simulink model "modelo_f_nico_local"  (R2024b)
settings: Solver=ode15s  StartTime=0.0  StopTime=600  FixedStep=0.001  RelTol=1e-3
InitFcn:
  | clc
  | clear
  | close all
  | parametros
  | gain_CL
  | calculo_observador_carro
  | calculo_observador_izaje
values from neighbouring files (symbols this model uses):
  b_cx = 1e6    (= 1000000)    [parametros.m]
  b_cy = 1e7    (= 10000000)    [parametros.m]
  b_ha = -(J_hEq + (r_hd/(2*i_h))*m_l) * w_des_h*(1 + n_h + n_h^2) + b_hEq    [gain_CL.m]
  b_hb = 1e8    (= 100000000)    [parametros.m]
  b_hd = 8    [parametros.m]
  b_hm = 18    [parametros.m]
  b_t = 90    [parametros.m]
  b_ta = M_tEq*w_des_t*(1+n_t+n_t^2)-b_tEq    [gain_CL.m]
  b_tb = 5e6    (= 5000000)    [parametros.m]
  b_td = 1.8    [parametros.m]
  b_tm = 6    [parametros.m]
  b_tw = 3e3    (= 3000)    [parametros.m]
  b_wu = 150    [parametros.m]
  g = 9.80665    [parametros.m]
  H_c = 2.59    [parametros.m]
  i_h = 22    [parametros.m]
  i_t = 30    [parametros.m]
  J_hd_hEb = 3800    [parametros.m]
  J_hm_hb = 30    [parametros.m]
  J_td = 1200    [parametros.m]
  J_tm_tb = 7    [parametros.m]
  K_cy = 1.8e9    (= 1800000000)    [parametros.m]
  k_hsa = -(J_hEq + (r_hd/(2*i_h))*m_l) * w_des_h^2*(n_h + n_h^2 + n_h^3)    [gain_CL.m]
  k_hsia = -(J_hEq + (r_hd/(2*i_h))*m_l) * n_h^3 * w_des_h^3    [gain_CL.m]
  k_tsa = M_tEq*w_des_t^2*n_t*(1+n_t+n_t^2)    [gain_CL.m]
  k_tsia = M_tEq*w_des_t^3*n_t^3    [gain_CL.m]
  K_tw = 4.8e5    (= 480000)    [parametros.m]
  k_wu = 2.36e8    (= 236000000)    [parametros.m]
  l_h_max = Y_t0-y_h_min    (= 65)    [parametros.m]
  l_h_maxE = l_h_max+0.5    (= 65.5)    [parametros.m]
  l_h_min = Y_t0-y_h_max    (= 5)    [parametros.m]
  l_h_minE = l_h_min-0.5    (= 4.5)    [parametros.m]
  Lt = place(At', Ct', polos_deseados)'    [calculo_observador_carro.m]
  M_cmax = 50000    [parametros.m]
  M_cmin = 2000    [parametros.m]
  M_s = 15000    [parametros.m]
  M_t = 30000    [parametros.m]
  r_hd = 0.75    [parametros.m]
  r_td = 0.50    (= 0.5)    [parametros.m]
  T_hbMax = 5e4    (= 50000)    [parametros.m]
  T_hEbMax = 1.1e6    (= 1100000)    [parametros.m]
  T_hmMax = 2e4    (= 20000)    [parametros.m]
  T_s = 0.001    [parametros.m]
  T_tbMax = 5e3    (= 5000)    [parametros.m]
  T_tmMax = 4e3    (= 4000)    [parametros.m]
  tau_tm = 1e-3    (= 0.001)    [parametros.m]
  tau_wl = 1 / (2 * pi * 2)    (= 0.0795774715459)    [parametros.m]
  theta_hm0 = -l_h0*i_h*2/r_hd    (= -2229.33333333)    [parametros.m]
  theta_tm0 = (x_t0)*i_t/r_td    (= -900)    [parametros.m]
  v_h_max_noload = 3    [parametros.m]
  v_lx0 = 0    [parametros.m]
  v_ly0 = 0    [parametros.m]
  v_t0 = 0    [parametros.m]
  v_t_max = 4    [parametros.m]
  W_c = ctrb(A, B_c(:,1))    [CyO_carro.m]    (also in CyO_izaje.m; parametros.m = 2.44)
  w_hm0 = 0    [parametros.m]
  w_hm_min_BRK = 999999999    [parametros.m]
  w_hm_rated = v_h_max_load*2*i_h/r_hd    (= 88)    [parametros.m]
  w_tm0 = (v_t0)*i_t/r_td    (= 0)    [parametros.m]
  w_tm_min_BRK = 999999999    [parametros.m]
  x_l0 = x_t0    (= -15)    [parametros.m]
  x_lidar_offset = 3.0    (= 3)    [parametros.m]
  x_t0 = -15    [parametros.m]
  x_t_max = 50    [parametros.m]
  x_t_maxE = x_t_max+0.5    (= 50.5)    [parametros.m]
  x_t_min = -30    [parametros.m]
  x_t_minE = x_t_min-0.5    (= -30.5)    [parametros.m]
  y_h_min = -20    [parametros.m]
  y_l0 = 7    [parametros.m]
  Y_sb = 5.0    (= 5)    [parametros.m]
  Y_t0 = 45    [parametros.m]
undefined symbols (not defined in the file or in its folder): carro_FC_safety_margin, izaje_FC_safety_margin, Lh
libraries: dspsigops x1, simulink x1
(part 2 of 2)

== system modelo_f_nico_local/Nivel 2/Subsistema físico/Carga/F_cy ==
  y_l : Inport
  v_ly : Inport  Port=2
  h_c : Inport  Port=3
  y_c0 : Inport  Port=4
  Constant1 : Constant  Value=0
  Gain : Gain  Gain=K_cy
  Gain1 : Gain  Gain=b_cy
  Sum : Sum  Inputs=|+-
  Sum1 : Sum  Inputs=|-+
  Sum2 : Sum  Inputs=|+-
  Sum3 : Sum  Inputs=|-+
  switch : Switch  Criteria=u2 > Threshold  SaturateOnIntegerOverflow=off  InputSameDT=off
  F_cy : Outport
  wires:
  switch/1 -> F_cy/1
  Sum2/1 -> switch/1
  Constant1/1 -> switch/3
  Sum/1 -> Sum3/1, Sum1/1
  y_l/1 -> Sum/1
  h_c/1 -> Sum/2
  y_c0/1 -> Sum3/2, Sum1/2
  Sum1/1 -> Gain/1
  Gain/1 -> Sum2/1
  v_ly/1 -> Gain1/1
  Gain1/1 -> Sum2/2
  Sum3/1 -> switch/2

== matlab function modelo_f_nico_local/Nivel 2/Subsistema físico/MATLAB Function1 ==
  data: y_lidar input; x_act input; x_target input; x_lidar_offset input; y_safe output; x_t_min input; x_t_max input; W_c input; y_h_min input; x_obs output
function [y_safe, x_obs] = gestor_memoria(y_lidar, x_act, x_target, x_lidar_offset, x_t_min, x_t_max, W_c, y_h_min)
% El Gemelo Digital: Construye el mapa cruzando datos
persistent x_grid memoria_mapa

%% 1. Creación de la memoria vacía
if isempty(memoria_mapa)
    x_grid = x_t_min : W_c : x_t_max;
    % Empieza asumiendo que todo es un foso profundo (y_h_min)
    memoria_mapa = ones(1, length(x_grid)) * y_h_min;
end

%% 2. GRABACIÓN EN VIVO (SLAM)
% El cerebro calcula dónde está mirando el sensor realmente
x_laser_calculado = x_act + x_lidar_offset;
x_laser_calculado = max(x_t_min, min(x_laser_calculado, x_t_max));

[~, idx_laser] = min(abs(x_grid - x_laser_calculado));

% Guardamos el dato 'y' ciego en la coordenada 'x' que calculamos
memoria_mapa(idx_laser) = y_lidar;

%% 3. EL ORÁCULO: Consulta de la ruta predictiva
[~, idx_act] = min(abs(x_grid - x_act));
[~, idx_target] = min(abs(x_grid - x_target));

idx_min = min(idx_act, idx_target);
idx_max = max(idx_act, idx_target);

% Exportamos el obstáculo más alto guardado en esa ventana espacial
[max_y_val, idx_max_local] = max(memoria_mapa(idx_min : idx_max));

H_c = 2.59;       % Altura del contenedor a levantar
margen_y = 2.0;   % Margen de seguridad vertical extra

% Devolvemos la altura segura final y la coordenada X de ese obstáculo
y_safe = max_y_val + H_c + margen_y;
x_obs = x_grid(idx_min + idx_max_local - 1);

end

== matlab function modelo_f_nico_local/Nivel 2/Controlador de Balanceo/MATLAB Function ==
  data: theta_l input; v_balanceo output; omega_l input; l input; dl_dt input; g input
function v_balanceo = controlador_balanceo(theta_l, omega_l, l, dl_dt, g)
    DEG2RAD = pi / 180;
    THRESH_V   = 0.05;
    THRESH_ACC = 0.1;

    if abs(omega_l) > THRESH_ACC
        theta_lim  = 15 * DEG2RAD;
        theta_full = 20 * DEG2RAD;
    elseif abs(omega_l) > THRESH_V
        theta_lim  = 3.5 * DEG2RAD;
        theta_full = 5   * DEG2RAD;
    else
        theta_lim  = 0;
        theta_full = 1   * DEG2RAD;
    end

    theta_margen = theta_full - theta_lim;
    abs_theta = abs(theta_l);
    if abs_theta >= theta_full
        escala = 1.0;
    elseif abs_theta > theta_lim
        escala = 0.5 + 0.5 * (abs_theta - theta_lim) / theta_margen;
    else
        escala = 0.0;
    end

    l_seg  = max(l, 0.1);
    th_sat = max(-80*DEG2RAD, min(80*DEG2RAD, theta_l));
    w_o    = sqrt(g / l_seg);
    K_do   = (2*w_o*l_seg - 2*dl_dt) / cos(th_sat);

    v_balanceo = escala * K_do * theta_l;
end

== matlab function modelo_f_nico_local/Nivel 2/Subsistema físico/MATLAB Function ==
  data: x_t_min input; y_c0_contacto output; x_t_max input; Y_sb input; W_c input; y_h_min input; H_c input; x_lidar_offset input; x_l input; TLK input; y_c0_lidar output
function [y_c0_contacto, y_c0_lidar] = perfil_suelo(x_t_min, x_t_max, Y_sb, W_c, y_h_min, H_c, x_lidar_offset, x_l, TLK)
% El Universo Físico: Simula la realidad y los sensores
persistent n_containers x_grid tlk_prev y_base_grid

%% 1. Inicialización de la física (Solo corre en t=0)
if isempty(n_containers)
    x_grid       = x_t_min : W_c : x_t_max;
    n_containers = zeros(1, length(x_grid));
    tlk_prev     = false;
    
    y_base_grid = zeros(1, length(x_grid));
    for i = 1:length(x_grid)
        if x_grid(i) < -W_c/2
            y_base_grid(i) = 0;
        elseif x_grid(i) >= -W_c/2 && x_grid(i) <= W_c/2
            y_base_grid(i) = Y_sb;
        else
            y_base_grid(i) = y_h_min;
        end
    end
end

%% Lectura de Sensores (Realidad actual)
y_total_grid = y_base_grid + (n_containers * H_c);

% Sensor 1: Altura física debajo del gancho
[~, idx_act] = min(abs(x_grid - x_l));
% --- NUEVA LÓGICA DE APILADO / DESAPILADO ---
% Detectamos los flancos de la señal TLK
flanco_subida = (tlk_prev == false) && (TLK == true);  % Toma carga
flanco_bajada = (tlk_prev == true)  && (TLK == false); % Deja carga

if flanco_subida
    % Si toma un contenedor, restamos 1 a esa posición (mínimo 0)
    n_containers(idx_act) = max(0, n_containers(idx_act) - 1);
elseif flanco_bajada
    % Si suelta un contenedor, sumamos 1 a esa posición
    n_containers(idx_act) = n_containers(idx_act) + 1;
end

% Actualizamos la memoria del estado anterior
tlk_prev = TLK;
% --------------------------------------------

% Calculamos la topografía actualizada
y_total_grid = y_base_grid + (n_containers * H_c);

% Sensor 1: Altura física debajo del gancho
y_c0_contacto = y_total_grid(idx_act);

% Sensor 2: SIMULACIÓN DEL LIDAR
x_laser = x_l + x_lidar_offset; % Calculamos dónde pega el rayo físico

% Protegemos para que no lea fuera del galpón
x_laser = max(x_t_min, min(x_laser, x_t_max));

[~, idx_lidar] = min(abs(x_grid - x_laser));
y_c0_lidar = y_total_grid(idx_lidar); % ¡Esta es la única salida real del sensor!
end

== stateflow chart modelo_f_nico_local/Chart ==
  settings: updateMethod=DISCRETE  sampleTime=0.02
  state Supervisory_Control
    state ON
      state BRK_Logic [parallel]
        settings: executionOrder=1
        state BRK_t_Logic [parallel]
          settings: executionOrder=1
          state BRK_t_Closed
            entry:
            BRK_t = false;
          state BRK_t_Opened
            entry:
            BRK_t = true;
          (default) -> BRK_t_Closed
          BRK_t_Opened -> BRK_t_Closed : [(~cmd_BRK_t && abs(w_tm_estimada) < w_tm_min_BRK) || FC_carro_min || FC_carro_max]
          BRK_t_Closed -> BRK_t_Opened : [cmd_BRK_t && ~(FC_carro_max || FC_carro_min)]
        state BRK_h_Logic [parallel]
          settings: executionOrder=2
          state BRK_h_Closed
            entry:
            BRK_h = false;
          state BRK_h_Opened
            entry:
            BRK_h = true;
          (default) -> BRK_h_Closed
          BRK_h_Opened -> BRK_h_Closed : [(~cmd_BRK_h && abs(w_hm_estimada) < w_hm_min_BRK) || FC_izaje_min || FC_izaje_max]
          BRK_h_Closed -> BRK_h_Opened : [cmd_BRK_h && ~(FC_izaje_max || FC_izaje_min)]
      state TLK_Logic [parallel]
        settings: executionOrder=2
        state Init
        state TLK_Opened
          entry:
          TLK = false;
        state TLK_Closed
          entry:
          TLK = true;
        (default) -> Init
        Init -> TLK_Closed [order 1] : [TLK]
        Init -> TLK_Opened [order 2] : [~TLK]
        TLK_Opened -> TLK_Closed : [cmd_TLK && abs(F_hw_sensor) <= 0]
        TLK_Closed -> TLK_Opened : [~cmd_TLK && abs(F_hw_sensor) <= 0]
      state Sway_Control_Mode [parallel]
        settings: executionOrder=3
        state Sway_Control_ON
          entry:
          sway_ctr_enable = true;
        state Sway_Control_OFF
          entry:
          sway_ctr_enable = false;
        (default) -> Sway_Control_ON
        Sway_Control_ON -> Sway_Control_OFF : [~cmd_sway_ctr]
        Sway_Control_OFF -> Sway_Control_ON : [cmd_sway_ctr && operation_mode == false]
      state Heartbeat_Generator [parallel]
        settings: executionOrder=4
        state Heartbeat_High
          entry:
          heartbeat = true;
        state Heartbeat_Low
          entry:
          heartbeat = false;
        (default) -> Heartbeat_High
        Heartbeat_Low -> Heartbeat_High : after(200, msec)
        Heartbeat_High -> Heartbeat_Low : after(200, msec)
      state Limit_Switch [parallel]
        during:
        force_manual_mode = FC_t_min_alarm || FC_t_max_alarm || FC_h_min_alarm || FC_h_max_alarm;
        settings: executionOrder=5
        state Trolley_Min_Logic [parallel]
          settings: executionOrder=1
          state FC_t_Min_High
            entry:
            FC_t_min_alarm = true;
          state FC_t_Min_Low
            entry:
            FC_t_min_alarm = false;
          (default) -> FC_t_Min_Low
          FC_t_Min_Low -> FC_t_Min_High : [FC_carro_min]
          FC_t_Min_High -> FC_t_Min_Low : [cmd_carro_FC_ack && x_td_sensor >= x_t_min + carro_FC_safety_margin]
        state Trolley_Max_Logic [parallel]
          settings: executionOrder=2
          state FC_t_Max_High
            entry:
            FC_t_max_alarm = true;
          state FC_t_Max_Low
            entry:
            FC_t_max_alarm = false;
          (default) -> FC_t_Max_Low
          FC_t_Max_Low -> FC_t_Max_High : [FC_carro_max]
          FC_t_Max_High -> FC_t_Max_Low : [cmd_carro_FC_ack && x_td_sensor <= x_t_max - carro_FC_safety_margin]
        state Hoist_Min_Logic [parallel]
          settings: executionOrder=3
          state FC_h_Min_High
            entry:
            FC_h_min_alarm = true;
            dl_h_ref = 0;
          state FC_h_Min_Low
            entry:
            FC_h_min_alarm = false;
          (default) -> FC_h_Min_Low
          FC_h_Min_Low -> FC_h_Min_High : [FC_izaje_min]
          FC_h_Min_High -> FC_h_Min_Low : [cmd_izaje_FC_ack && l_h_sensor >= l_h_minE + izaje_FC_safety_margin]
        state Hoist_Max_Logic [parallel]
          settings: executionOrder=4
          state FC_h_Max_Low
            entry:
            FC_h_max_alarm = false;
          state FC_h_Max_High
            entry:
            FC_h_max_alarm = true;
          (default) -> FC_h_Max_Low
          FC_h_Max_Low -> FC_h_Max_High : [FC_izaje_max]
          FC_h_Max_High -> FC_h_Max_Low : [cmd_izaje_FC_ack && l_h_sensor <= l_h_max - izaje_FC_safety_margin]
      state Lidar_Map [parallel]
        entry:
        mapa_y(:) = 0;
        during:
        % 1. Sumamos el offset del lidar para saber dónde mira realmente el láser
        x_laser = x_td_sensor + 3.0;
        % 2. Convertimos a índice (resolución 0.01m, arrancando desde x_t_min = -30)
        x_idx = round((x_laser - (-30.0)) / 0.01) + 1;
        % 3. Protegemos contra desbordamientos del arreglo
        x_idx = max(1, min(length(mapa_y), x_idx));
        % 4. Guardamos la altura en esa coordenada exacta
        mapa_y(x_idx) = y_c0_lidar;
        settings: executionOrder=6
      state Mode [parallel]
        settings: executionOrder=7
        state Manual
          entry:
          operation_mode = false;
          during:
          x_target = x_act;
          y_target = y_act;
        state Mapping
          entry:
          operation_mode = true;
          exit:
          mapa_listo = true;
          state Subir_Carga
            entry:
            x_target = x_act;
            y_target = 25.0;
          state Ida
            entry:
            x_target = 50.0;
            y_target = 25.0;
          state Vuelta
            entry:
            x_target = -30.0;
            y_target = 25;
          (default) -> Subir_Carga
          Subir_Carga -> Ida : [y_act >= 24.2]
          Ida -> Vuelta : [x_act >= 49.5 && (abs(v_act) <= 0.5)]
        state Ciclo_Operativo
          state Pensar_Ruta
            entry:
            operation_mode = false;
            x_target = 40.0
          state Escape_y_Traslacion
            entry:
            operation_mode = true;
            y_target = y_safe;
          state Aproximacion_Final
            entry:
            y_target = 0.0;
          (default) -> Pensar_Ruta
          Pensar_Ruta -> Escape_y_Traslacion : [after(0.1, sec)]
          Escape_y_Traslacion -> Aproximacion_Final : [abs(x_target - x_act) <= abs(x_target - x_obs)]
        (default) -> Manual : {operation_mode = false;}
        Aproximacion_Final -> Manual : [abs(x_target - x_act) < 0.1 && abs(y_target - y_act) < 0.1 && abs(v_act) < 0.1]
        Manual -> Ciclo_Operativo [order 2] : [start_auto && mapa_listo]
        Vuelta -> Manual : [x_act <= -29.5 && abs(v_act) <= 0.5]
        Manual -> Mapping [order 1] : [[start_mapping && ~mapa_listo]]
    state OFF
      entry:
      BRK_h = false;
      BRK_t = false;
      TLK = false;
      v_t_ref = 0.0;
      dl_h_ref = 0.0;
      sway_ctr_enable = false;
      FC_t_min_alarm = false;
      FC_t_max_alarm = false;
      FC_h_min_alarm = false;
      FC_h_max_alarm = false;
      force_manual_mode = false;
      sway_ctr_enable = false;
      heartbeat = false;
      operation_mode = false;
    (default) -> OFF
    OFF -> ON : [P_APN]
    ON -> OFF : [~P_APN]
  (default) -> Supervisory_Control
  data: FCE_izaje_min input boolean size=1; BRK_t output boolean size=1; v_t_ref output double size=1; cmd_TLK output; BRK_h output boolean size=1; x_td_sensor input; theta_tm_sensor input; l_h_sensor input; theta_hm_sensor input; theta_l_sensor input; w_l_sensor input; w_tm_estimada input; w_hm_estimada input; y_c0_lidar input; P_APN input; P_E input boolean; cmd_carro_FC_ack input; cmd_sway_ctr input; cmd_izaje_FC_ack input; FCE_carro_min input boolean; FCE_carro_max input boolean size=1; FC_izaje_min input; FC_izaje_max input; FCE_izaje_max input boolean; sobrevelocidad_carro input; sobrevelocidad_izaje_noload input; FC_carro_max input; FC_carro_min input; cmd_TLK input; cmd_BRK_h input; cmd_BRK_t input; F_hw_sensor input; w_hm_min_BRK parameter; w_tm_min_BRK parameter; sway_ctr_enable output boolean size=1; dl_h_ref output double size=1; FC_h_max_alarm local; FC_h_min_alarm local; FC_t_max_alarm local; FC_t_min_alarm local; TLK local; dx_grid local; force_manual_mode local; n_grid local; x_idx local; heartbeat output boolean size=1; izaje_FC_safety_margin parameter; carro_FC_safety_margin parameter; l_h_max parameter; x_t_max parameter; x_t_min parameter; l_h_minE parameter; mapa_y output double size=LIDAR_GRID_SIZE; operation_mode output boolean =false; x_target output double size=1; y_target output double size=1; x_laser local; x_act input; y_act input; start_mapping input boolean size=1; start_auto input boolean size=1; v_t_scan local; v_h_up local; v_act input double; y_safe input; mapa_listo local boolean =false; x_obs input

== matlab function modelo_f_nico_local/MATLAB Function4 ==
  data: x_target input; x_ref output; x_act input; v_act input; enable input; v_ref output; a_ref output
function [x_ref, v_ref, a_ref] = generador_carro(x_target, x_act, v_act, enable)
    % PARÁMETROS FÍSICOS DEL CARRO
    v_max = 4.0; % [m/s]
    a_max = 0.8; % [m/s^2]
    Ts = 0.001;  % [s]
    
    % MEMORIA DEL GENERADOR
    persistent enable_prev x_r v_r
    if isempty(enable_prev)
        enable_prev = false;
        x_r = 0; 
        v_r = 0;
    end
    
    if enable == false
        % --- MODO MANUAL / FRENO ---
        x_r = x_act;
        v_r = 0;
        a_ref = 0;
    else
        % --- MODO AUTOMÁTICO ---
        if enable_prev == false
            % Flanco de subida: Bumpless transfer perfecto
            x_r = x_act;
            v_r = v_act;
        end
        
        % Control cinemático paso a paso
        error = x_target - x_r;
        dir = sign(error);
        dist = abs(error);
        
        % 1. Raíz cuadrada para perfil de frenado óptimo
        v_permitida = sqrt(2 * a_max * dist);
        v_obj = min(v_max, v_permitida) * dir;
        
        % 2. Control de aceleración para alcanzar v_obj
        error_v = v_obj - v_r;
        if abs(error_v) > (a_max * Ts)
            a_ref = sign(error_v) * a_max;
        else
            a_ref = error_v / Ts; % Clava la velocidad exacta en el último step
        end
        
        % 3. LLEGADA: Enclavamiento suave
        if dist < 0.01 && abs(v_r) < 0.01
            x_r = x_target;
            v_r = 0;
            a_ref = 0;
        else
            % Integración numérica de la trayectoria teórica
            v_r = v_r + a_ref * Ts;
            x_r = x_r + v_r * Ts;
        end
    end
    
    enable_prev = enable;
    
    % ASIGNACIÓN DE SALIDAS
    x_ref = x_r;
    
    % Recuperación final para el PID del Nivel 2
    if enable && (abs(x_target - x_r) < 0.01)
        v_ref = 0.2 * (x_target - x_act); 
    else
        v_ref = v_r;
    end
end

== matlab function modelo_f_nico_local/MATLAB Function5 ==
  data: x_target input; x_ref output; x_act input; v_act input; enable input; v_ref output; a_ref output
function [x_ref, v_ref, a_ref] = generador_izaje(x_target, x_act, v_act, enable)
    % PARÁMETROS FÍSICOS DEL IZAJE
    v_max = 3.0; % [m/s] Límite de velocidad
    a_max = 0.75; % [m/s^2] Límite de aceleración
    Ts = 0.001;  % [s] Tiempo de muestreo (1 ms)
    
    % MEMORIA DEL BLOQUE 
    persistent t_auto       
    persistent x0 v0        
    persistent dir          
    persistent ta tc td     
    persistent t1 t2 t3       
    persistent v_alcanzada    
    persistent calculo_ok   
    persistent meta_anterior 
    
    % Inicialización
    if isempty(t_auto)
        t_auto = 0; calculo_ok = false;
        x0 = 0; v0 = 0; dir = 1;
        ta = 0; tc = 0; td = 0;
        t1 = 0; t2 = 0; t3 = 0;       
        v_alcanzada = 0;              
        meta_anterior = x_target; 
    end
    
    if meta_anterior ~= x_target
        calculo_ok = false;
        t_auto = 0;
        meta_anterior = x_target;
    end
    
    %% MÁQUINA DE ESTADOS DEL GENERADOR
    if enable == false
        % --- MODO MANUAL (Freno de Seguridad) ---
        x_ref = x_act;
        v_ref = 0.0;   % CORRECCIÓN: Velocidad estrictamente cero
        a_ref = 0.0;
        t_auto = 0;           
        calculo_ok = false;
        return;        % CORRECCIÓN: Corta la ejecución acá mismo
    else
        % --- MODO AUTOMÁTICO (PERFIL TRAPEZOIDAL RÁPIDO) ---
        if calculo_ok == false
            x0 = x_act;       
            v0 = -v_act; % Traducción al idioma del motor
            
            D = x_target - x0; 
            dir = sign(D);     
            if dir == 0, dir = 1; end 
            dist = abs(D);     
            
            dist_acel = abs(v_max^2 - v0^2) / (2 * a_max); 
            dist_freno = (v_max^2) / (2 * a_max); 
            
            if dist >= (dist_acel + dist_freno)
                ta = (v_max - abs(v0)) / a_max;                  
                td = v_max / a_max;                            
                dist_constante = dist - (dist_acel + dist_freno); 
                tc = dist_constante / v_max;         
                v_alcanzada = v_max;                 
            else
                v_alcanzada = sqrt((2 * a_max * dist + v0^2) / 2); 
                ta = (v_alcanzada - abs(v0)) / a_max;
                td = v_alcanzada / a_max; 
                tc = 0; 
            end
            
            t1 = ta;           
            t2 = ta + tc;      
            t3 = ta + tc + td; 
            calculo_ok = true; 
        end
        
        t_auto = t_auto + Ts; 
        
        if t_auto <= t1
            a_ref = dir * a_max;
            v_ref = v0 + (a_ref * t_auto);
            x_ref = x0 + (v0 * t_auto) + (0.5 * a_ref * t_auto^2);
        elseif t_auto <= t2
            a_ref = 0;
            v_ref = dir * v_alcanzada;
            dist_fase1 = abs(v0 * t1 + 0.5 * (dir * a_max) * t1^2); 
            tiempo_en_fase2 = (t_auto - t1);
            x_ref = x0 + dir * (dist_fase1 + v_alcanzada * tiempo_en_fase2);
        elseif t_auto <= t3
            a_ref = -dir * a_max;
            tiempo_en_fase3 = (t_auto - t2);
            v_ref = dir * (v_alcanzada - a_max * tiempo_en_fase3);
            dist_fase1 = abs(v0 * t1 + 0.5 * (dir * a_max) * t1^2); 
            dist_fase2 = v_alcanzada * tc;
            dist_fase3 = v_alcanzada * tiempo_en_fase3 - 0.5 * a_max * tiempo_en_fase3^2;
            x_ref = x0 + dir * (dist_fase1 + dist_fase2 + dist_fase3);
        else
            a_ref = 0;
            v_ref = 0;
            x_ref = x_target; 
        end
        
        % Traducción final para el motor
        v_ref = -v_ref;
        a_ref = -a_ref;
    end
end

== matlab function modelo_f_nico_local/MATLAB Function6 ==
  data: enable_izaje output; enable_auto input; enable_carro output; x_act input; y_act input; x_obs input; y_safe input
function [enable_izaje, enable_carro] = coordinador_trayectorias(enable_auto, x_act, y_act, x_obs, y_safe)
    
    % --- FORZADO DE ESCALARES PARA EL COMPILADOR ---
    % Garantiza que Simulink los trate como números 1x1
    x_act  = x_act(1);
    y_act  = y_act(1);
    x_obs  = x_obs(1);
    y_safe = y_safe(1);
    % -----------------------------------------------

    % PARÁMETROS FÍSICOS
    v_max_t = 4.0;
    a_max_t = 0.8;
    v_max_h = 3.0;
    
    % MEMORIA DEL BLOQUE
    persistent carro_liberado
    
    if isempty(carro_liberado)
        carro_liberado = false;
    end
    
    if enable_auto == false
        % --- REPOSO / MODO MANUAL ---
        enable_carro = false;
        enable_izaje = false;
        carro_liberado = false;
        return;
    end
    
    % LÓGICA DE RETENCIÓN (Semáforo)
    enable_izaje = true; % El izaje siempre arranca primero para escapar
    
    if carro_liberado == true
        enable_carro = true;
    else
        % Cinemática para saber si liberar el carro
        dist_obs = abs(x_obs - x_act);
        dist_acel_carro = (v_max_t^2) / (2 * a_max_t);
        
        if dist_obs >= dist_acel_carro
            t_impacto = (v_max_t / a_max_t) + (dist_obs - dist_acel_carro) / v_max_t;
        else
            t_impacto = sqrt(2 * dist_obs / a_max_t);
        end
        
        dist_y_faltante = y_safe - y_act;
        if dist_y_faltante <= 0
            t_escape = 0; 
        else
            t_escape = dist_y_faltante / v_max_h; 
        end
        
        margen_seguridad_s = 0.5; 
        
        if (t_impacto > t_escape + margen_seguridad_s) || (y_act >= y_safe)
            carro_liberado = true;
            enable_carro = true;
        else
            enable_carro = false; 
        end
    end
end
